simulink model "PID_quad_x_model"  (R2014b)
settings: Solver=ode45  StartTime=0.0  StopTime=30.0  RelTol=1e-3
libraries: simulink x5
settings Model: Creator=ghost  LastModifiedBy=ghost

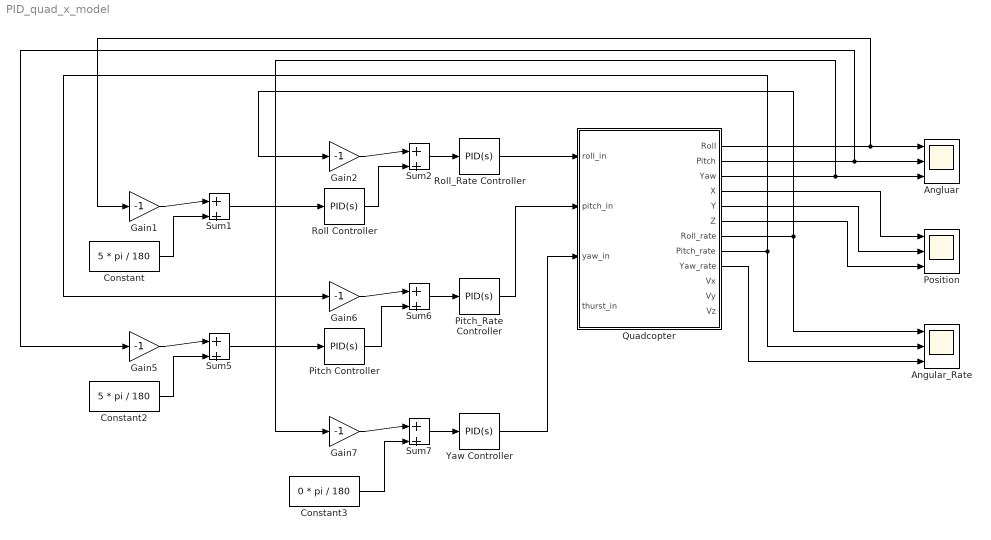
== system PID_quad_x_model ==
  Angluar : Scope  NumInputPorts=3
      settings: YMin=-5~-5~-5  YMax=5~5~5  SaveName=ScopeData2
  Angular_Rate : Scope  NumInputPorts=3
      settings: YMin=-5~-5~-5  YMax=5~5~5  SaveName=ScopeData3
  Constant : Constant  Value=5 * pi / 180
  Constant2 : Constant  Value=5 * pi / 180
  Constant3 : Constant  Value=0 * pi / 180
  Gain{1..2,5..7} (5 alike) : Gain  Gain=-1
  Pitch Controller : simulink/Continuous/PID Controller  Controller=PID  TimeDomain=Continuous-time  SampleTime=-1  IntegratorMethod=Forward Euler  FilterMethod=Forward Euler  Form=Parallel  P=10  I=0.05  D=0  N=100  InitialConditionSource=internal  InitialConditionForIntegrator=0  InitialConditionForFilter=0  ExternalReset=none  LimitOutput=off  UpperSaturationLimit=inf  LowerSaturationLimit=-inf  LinearizeAsGain=on  AntiWindupMode=none  Kb=1  TrackingMode=off  Kt=1  PParamMin=[]  PParamMax=[]  IParamMin=[]  IParamMax=[]  DParamMin=[]  DParamMax=[]  NParamMin=[]  NParamMax=[]  KbParamMin=[]  KbParamMax=[]  KtParamMin=[]  KtParamMax=[]  POutMin=[]  POutMax=[]  IOutMin=[]  IOutMax=[]  DOutMin=[]  DOutMax=[]  NOutMin=[]  NOutMax=[]  KbOutMin=[]  KbOutMax=[]  KtOutMin=[]  KtOutMax=[]  IntegratorOutMin=[]  IntegratorOutMax=[]  FilterOutMin=[]  FilterOutMax=[]  SumOutMin=[]  SumOutMax=[]  SumI1OutMin=[]  SumI1OutMax=[]  SumI2OutMin=[]  SumI2OutMax=[]  SumI3OutMin=[]  SumI3OutMax=[]  SumDOutMin=[]  SumDOutMax=[]  SaturationOutMin=[]  SaturationOutMax=[]  IntegratorContinuousStateAttributes=''  IntegratorStateMustResolveToSignalObject=off  IntegratorRTWStateStorageClass=Auto  FilterContinuousStateAttributes=''  FilterStateMustResolveToSignalObject=off  FilterRTWStateStorageClass=Auto  DifferentiatorICPrevScaledInput=0  DifferentiatorOutMin=[]  DifferentiatorOutMax=[]  UseFilter=on
  Pitch_Rate Controller : simulink/Continuous/PID Controller  Controller=PID  TimeDomain=Continuous-time  SampleTime=-1  IntegratorMethod=Forward Euler  FilterMethod=Forward Euler  Form=Parallel  P=1  I=0  D=0.1  N=100  InitialConditionSource=internal  InitialConditionForIntegrator=0  InitialConditionForFilter=0  ExternalReset=none  LimitOutput=off  UpperSaturationLimit=inf  LowerSaturationLimit=-inf  LinearizeAsGain=on  AntiWindupMode=none  Kb=1  TrackingMode=off  Kt=1  PParamMin=[]  PParamMax=[]  IParamMin=[]  IParamMax=[]  DParamMin=[]  DParamMax=[]  NParamMin=[]  NParamMax=[]  KbParamMin=[]  KbParamMax=[]  KtParamMin=[]  KtParamMax=[]  POutMin=[]  POutMax=[]  IOutMin=[]  IOutMax=[]  DOutMin=[]  DOutMax=[]  NOutMin=[]  NOutMax=[]  KbOutMin=[]  KbOutMax=[]  KtOutMin=[]  KtOutMax=[]  IntegratorOutMin=[]  IntegratorOutMax=[]  FilterOutMin=[]  FilterOutMax=[]  SumOutMin=[]  SumOutMax=[]  SumI1OutMin=[]  SumI1OutMax=[]  SumI2OutMin=[]  SumI2OutMax=[]  SumI3OutMin=[]  SumI3OutMax=[]  SumDOutMin=[]  SumDOutMax=[]  SaturationOutMin=[]  SaturationOutMax=[]  IntegratorContinuousStateAttributes=''  IntegratorStateMustResolveToSignalObject=off  IntegratorRTWStateStorageClass=Auto  FilterContinuousStateAttributes=''  FilterStateMustResolveToSignalObject=off  FilterRTWStateStorageClass=Auto  DifferentiatorICPrevScaledInput=0  DifferentiatorOutMin=[]  DifferentiatorOutMax=[]  UseFilter=on
  Position : Scope  NumInputPorts=3
      settings: YMin=-5~-5~-5  YMax=5~5~5  SaveName=ScopeData4
  Quadcopter : Subsystem
  Roll Controller : simulink/Continuous/PID Controller  Controller=PID  TimeDomain=Continuous-time  SampleTime=-1  IntegratorMethod=Forward Euler  FilterMethod=Forward Euler  Form=Parallel  P=10  I=0.05  D=0  N=100  InitialConditionSource=internal  InitialConditionForIntegrator=0  InitialConditionForFilter=0  ExternalReset=none  LimitOutput=off  UpperSaturationLimit=inf  LowerSaturationLimit=-inf  LinearizeAsGain=on  AntiWindupMode=none  Kb=1  TrackingMode=off  Kt=1  PParamMin=[]  PParamMax=[]  IParamMin=[]  IParamMax=[]  DParamMin=[]  DParamMax=[]  NParamMin=[]  NParamMax=[]  KbParamMin=[]  KbParamMax=[]  KtParamMin=[]  KtParamMax=[]  POutMin=[]  POutMax=[]  IOutMin=[]  IOutMax=[]  DOutMin=[]  DOutMax=[]  NOutMin=[]  NOutMax=[]  KbOutMin=[]  KbOutMax=[]  KtOutMin=[]  KtOutMax=[]  IntegratorOutMin=[]  IntegratorOutMax=[]  FilterOutMin=[]  FilterOutMax=[]  SumOutMin=[]  SumOutMax=[]  SumI1OutMin=[]  SumI1OutMax=[]  SumI2OutMin=[]  SumI2OutMax=[]  SumI3OutMin=[]  SumI3OutMax=[]  SumDOutMin=[]  SumDOutMax=[]  SaturationOutMin=[]  SaturationOutMax=[]  IntegratorContinuousStateAttributes=''  IntegratorStateMustResolveToSignalObject=off  IntegratorRTWStateStorageClass=Auto  FilterContinuousStateAttributes=''  FilterStateMustResolveToSignalObject=off  FilterRTWStateStorageClass=Auto  DifferentiatorICPrevScaledInput=0  DifferentiatorOutMin=[]  DifferentiatorOutMax=[]  UseFilter=on
  Roll_Rate Controller : simulink/Continuous/PID Controller  Controller=PID  TimeDomain=Continuous-time  SampleTime=-1  IntegratorMethod=Forward Euler  FilterMethod=Forward Euler  Form=Parallel  P=1  I=0  D=0.1  N=100  InitialConditionSource=internal  InitialConditionForIntegrator=0  InitialConditionForFilter=0  ExternalReset=none  LimitOutput=off  UpperSaturationLimit=inf  LowerSaturationLimit=-inf  LinearizeAsGain=on  AntiWindupMode=none  Kb=1  TrackingMode=off  Kt=1  PParamMin=[]  PParamMax=[]  IParamMin=[]  IParamMax=[]  DParamMin=[]  DParamMax=[]  NParamMin=[]  NParamMax=[]  KbParamMin=[]  KbParamMax=[]  KtParamMin=[]  KtParamMax=[]  POutMin=[]  POutMax=[]  IOutMin=[]  IOutMax=[]  DOutMin=[]  DOutMax=[]  NOutMin=[]  NOutMax=[]  KbOutMin=[]  KbOutMax=[]  KtOutMin=[]  KtOutMax=[]  IntegratorOutMin=[]  IntegratorOutMax=[]  FilterOutMin=[]  FilterOutMax=[]  SumOutMin=[]  SumOutMax=[]  SumI1OutMin=[]  SumI1OutMax=[]  SumI2OutMin=[]  SumI2OutMax=[]  SumI3OutMin=[]  SumI3OutMax=[]  SumDOutMin=[]  SumDOutMax=[]  SaturationOutMin=[]  SaturationOutMax=[]  IntegratorContinuousStateAttributes=''  IntegratorStateMustResolveToSignalObject=off  IntegratorRTWStateStorageClass=Auto  FilterContinuousStateAttributes=''  FilterStateMustResolveToSignalObject=off  FilterRTWStateStorageClass=Auto  DifferentiatorICPrevScaledInput=0  DifferentiatorOutMin=[]  DifferentiatorOutMax=[]  UseFilter=on
  Sum{1..2,5..7} (5 alike) : Sum  Inputs=|++
  Yaw Controller : simulink/Continuous/PID Controller  Controller=PID  TimeDomain=Continuous-time  SampleTime=-1  IntegratorMethod=Forward Euler  FilterMethod=Forward Euler  Form=Parallel  P=1  I=0  D=1.25  N=100  InitialConditionSource=internal  InitialConditionForIntegrator=0  InitialConditionForFilter=0  ExternalReset=none  LimitOutput=off  UpperSaturationLimit=inf  LowerSaturationLimit=-inf  LinearizeAsGain=on  AntiWindupMode=none  Kb=1  TrackingMode=off  Kt=1  PParamMin=[]  PParamMax=[]  IParamMin=[]  IParamMax=[]  DParamMin=[]  DParamMax=[]  NParamMin=[]  NParamMax=[]  KbParamMin=[]  KbParamMax=[]  KtParamMin=[]  KtParamMax=[]  POutMin=[]  POutMax=[]  IOutMin=[]  IOutMax=[]  DOutMin=[]  DOutMax=[]  NOutMin=[]  NOutMax=[]  KbOutMin=[]  KbOutMax=[]  KtOutMin=[]  KtOutMax=[]  IntegratorOutMin=[]  IntegratorOutMax=[]  FilterOutMin=[]  FilterOutMax=[]  SumOutMin=[]  SumOutMax=[]  SumI1OutMin=[]  SumI1OutMax=[]  SumI2OutMin=[]  SumI2OutMax=[]  SumI3OutMin=[]  SumI3OutMax=[]  SumDOutMin=[]  SumDOutMax=[]  SaturationOutMin=[]  SaturationOutMax=[]  IntegratorContinuousStateAttributes=''  IntegratorStateMustResolveToSignalObject=off  IntegratorRTWStateStorageClass=Auto  FilterContinuousStateAttributes=''  FilterStateMustResolveToSignalObject=off  FilterRTWStateStorageClass=Auto  DifferentiatorICPrevScaledInput=0  DifferentiatorOutMin=[]  DifferentiatorOutMax=[]  UseFilter=on
  wires:
  Sum1/1 -> Roll Controller/1
  Gain1/1 -> Sum1/1
  Constant/1 -> Sum1/2
  Roll_Rate Controller/1 -> Quadcopter/1(roll_in)
  Sum2/1 -> Roll_Rate Controller/1
  Gain2/1 -> Sum2/1
  Roll Controller/1 -> Sum2/2
  Quadcopter/7(Roll_rate) -> Angular_Rate/1, Gain2/1
  Quadcopter/1(Roll) -> Angluar/1, Gain1/1
  Quadcopter/2(Pitch) -> Angluar/2, Gain5/1
  Quadcopter/3(Yaw) -> Angluar/3, Gain7/1
  Sum5/1 -> Pitch Controller/1
  Gain5/1 -> Sum5/1
  Constant2/1 -> Sum5/2
  Sum6/1 -> Pitch_Rate Controller/1
  Gain6/1 -> Sum6/1
  Pitch Controller/1 -> Sum6/2
  Quadcopter/8(Pitch_rate) -> Angular_Rate/2, Gain6/1
  Pitch_Rate Controller/1 -> Quadcopter/2(pitch_in)
  Yaw Controller/1 -> Quadcopter/3(yaw_in)
  Sum7/1 -> Yaw Controller/1
  Gain7/1 -> Sum7/1
  Constant3/1 -> Sum7/2
  Quadcopter/9(Yaw_rate) -> Angular_Rate/3
  Quadcopter/4(X) -> Position/1
  Quadcopter/5(Y) -> Position/2
  Quadcopter/6(Z) -> Position/3

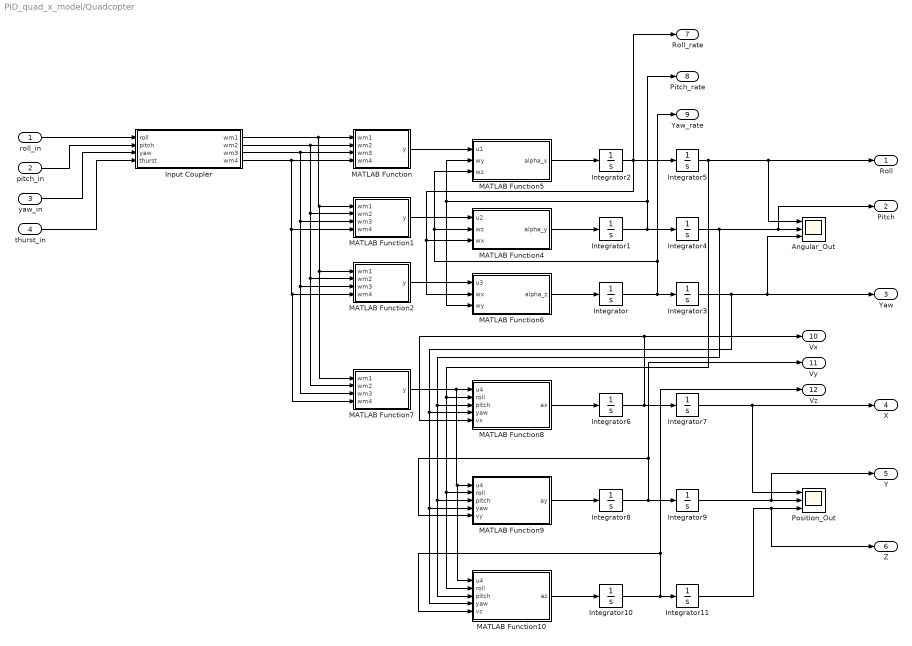
== system PID_quad_x_model/Quadcopter ==
  roll_in : Inport
  pitch_in : Inport  Port=2
  yaw_in : Inport  Port=3
  thurst_in : Inport  Port=4
  Angular_Out : Scope  NumInputPorts=3
      settings: YMin=-5~-5~-5  YMax=5~5~5
  Input Coupler : MATLAB Function  TreatAsAtomicUnit=on
  Integrator{,1..11} (12 alike) : Integrator
  MATLAB Function : MATLAB Function  TreatAsAtomicUnit=on
  MATLAB Function1 : MATLAB Function  TreatAsAtomicUnit=on
  MATLAB Function10 : MATLAB Function  TreatAsAtomicUnit=on
  MATLAB Function2 : MATLAB Function  TreatAsAtomicUnit=on
  MATLAB Function4 : MATLAB Function  TreatAsAtomicUnit=on
  MATLAB Function5 : MATLAB Function  TreatAsAtomicUnit=on
  MATLAB Function6 : MATLAB Function  TreatAsAtomicUnit=on
  MATLAB Function7 : MATLAB Function  TreatAsAtomicUnit=on
  MATLAB Function8 : MATLAB Function  TreatAsAtomicUnit=on
  MATLAB Function9 : MATLAB Function  TreatAsAtomicUnit=on
  "Position_Out " : Scope  NumInputPorts=3
      settings: YMin=-5~-5~-5  YMax=5~5~5
  Roll : Outport
  Pitch : Outport  Port=2
  Yaw : Outport  Port=3
  X : Outport  Port=4
  Y : Outport  Port=5
  Z : Outport  Port=6
  Roll_rate : Outport  Port=7
  Pitch_rate : Outport  Port=8
  Yaw_rate : Outport  Port=9
  Vx : Outport  Port=10
  Vy : Outport  Port=11
  Vz : Outport  Port=12
  wires:
  Input Coupler/1(wm1) -> MATLAB Function7/1(wm1), MATLAB Function2/1(wm1), MATLAB Function1/1(wm1), MATLAB Function/1(wm1)
  Input Coupler/2(wm2) -> MATLAB Function7/2(wm2), MATLAB Function2/2(wm2), MATLAB Function1/2(wm2), MATLAB Function/2(wm2)
  Input Coupler/3(wm3) -> MATLAB Function7/3(wm3), MATLAB Function2/3(wm3), MATLAB Function1/3(wm3), MATLAB Function/3(wm3)
  Input Coupler/4(wm4) -> MATLAB Function7/4(wm4), MATLAB Function2/4(wm4), MATLAB Function1/4(wm4), MATLAB Function/4(wm4)
  MATLAB Function1/1(y) -> MATLAB Function4/1(u2)
  MATLAB Function2/1(y) -> MATLAB Function6/1(u3)
  MATLAB Function6/1(alpha_z) -> Integrator/1
  Integrator/1 -> Integrator3/1, Yaw_rate/1, MATLAB Function5/3(wz), MATLAB Function4/2(wz)
  MATLAB Function5/1(alpha_x) -> Integrator2/1
  MATLAB Function4/1(alpha_y) -> Integrator1/1
  Integrator2/1 -> Integrator5/1, Roll_rate/1, MATLAB Function6/2(wx), MATLAB Function4/3(wx)
  Integrator3/1 -> MATLAB Function10/4(yaw), MATLAB Function9/4(yaw), MATLAB Function8/4(yaw), Yaw/1, Angular_Out/3
  Integrator4/1 -> Pitch/1, Angular_Out/2, MATLAB Function10/3(pitch), MATLAB Function9/3(pitch), MATLAB Function8/3(pitch)
  MATLAB Function/1(y) -> MATLAB Function5/1(u1)
  MATLAB Function8/1(ax) -> Integrator6/1
  Integrator6/1 -> Vx/1, MATLAB Function8/5(vx), Integrator7/1
  MATLAB Function7/1(y) -> MATLAB Function10/1(u4), MATLAB Function9/1(u4), MATLAB Function8/1(u4)
  MATLAB Function9/1(ay) -> Integrator8/1
  Integrator8/1 -> Vy/1, MATLAB Function9/5(vy), Integrator9/1
  MATLAB Function10/1(az) -> Integrator10/1
  Integrator5/1 -> MATLAB Function10/2(roll), MATLAB Function9/2(roll), MATLAB Function8/2(roll), Roll/1, Angular_Out/1
  Integrator7/1 -> X/1, "Position_Out "/1
  Integrator9/1 -> Y/1, "Position_Out "/2
  Integrator11/1 -> Z/1, "Position_Out "/3
  roll_in/1 -> Input Coupler/1(roll)
  pitch_in/1 -> Input Coupler/2(pitch)
  yaw_in/1 -> Input Coupler/3(yaw)
  thurst_in/1 -> Input Coupler/4(thurst)
  Integrator1/1 -> Pitch_rate/1, MATLAB Function5/2(wy), MATLAB Function6/3(wy), Integrator4/1
  Integrator10/1 -> Vz/1, MATLAB Function10/5(vz), Integrator11/1

== matlab function PID_quad_x_model/Quadcopter/MATLAB Function1 ==
  data: wm1 input; y output; wm2 input; wm3 input; wm4 input
function y = u2(wm1, wm2, wm3, wm4)
%#codegen

k1 = 3.1 * 10^-7;
y = k1 * (wm2^2 + wm4^2 - wm1^2 - wm3^2);
return;

== matlab function PID_quad_x_model/Quadcopter/MATLAB Function ==
  data: wm1 input; y output; wm2 input; wm3 input; wm4 input
function y = u1(wm1, wm2, wm3, wm4)
%#codegen

k1 = 3.1 * 10^-7;
y = k1 * (wm2^2 + wm3^2 - wm1^2 - wm4^2);
return;

== matlab function PID_quad_x_model/Quadcopter/MATLAB Function2 ==
  data: wm1 input; y output; wm2 input; wm3 input; wm4 input
function y = u3(wm1, wm2, wm3, wm4)
%#codegen

k2 = 3.1 * 10^-7;
y = k2 * (wm1^2 + wm2^2 - wm3^2 - wm4^2);
return;

== matlab function PID_quad_x_model/Quadcopter/Input Coupler ==
  data: roll input; wm1 output; pitch input; yaw input; thurst input; wm2 output; wm3 output; wm4 output
function [wm1, wm2, wm3, wm4] = input_coupler(roll, pitch, yaw, thurst)
%#codegen

% 控制耦合
% 输入是归一化的，-1~1

% 基础输入 1000
thurst_bias = 1407;

% 去归一化
roll  = roll  * 500;
pitch = pitch * 500;
yaw   = yaw   * 500;
thurst = thurst * 1000;

wm1 = thurst + thurst_bias - roll - pitch + yaw;
wm2 = thurst + thurst_bias + roll + pitch + yaw;
wm3 = thurst + thurst_bias + roll - pitch - yaw;
wm4 = thurst + thurst_bias - roll + pitch - yaw;


return;

== matlab function PID_quad_x_model/Quadcopter/MATLAB Function4 ==
  data: u2 input; wz input; alpha_y output; wx input
function alpha_y = calc_pitch_a(u2, wz, wx)
%#codegen

l = 0.25;
Jx = 0.033;
Jy = 0.033;
Jz = 0.061;

alpha_y = u2 * (sqrt(2) / 2) * l + (Jz - Jx) * wz * wx;
alpha_y = alpha_y / Jy;


return;

== matlab function PID_quad_x_model/Quadcopter/MATLAB Function5 ==
  data: u1 input; wy input; wz input; alpha_x output
function alpha_x = calc_roll_a(u1, wy, wz)
%#codegen

l = 0.25;
Jx = 0.033;
Jy = 0.033;
Jz = 0.061;

alpha_x = u1 * (sqrt(2) / 2) * l + (Jy - Jz) * wy * wz;
alpha_x = alpha_x / Jx;


return;

== matlab function PID_quad_x_model/Quadcopter/MATLAB Function6 ==
  data: u3 input; wx input; alpha_z output; wy input
function alpha_z = calc_yaw_a(u3, wx, wy)
%#codegen

l = 0.25;
Jx = 0.033;
Jy = 0.033;
Jz = 0.061;

alpha_z = u3 * l + (Jx - Jy) * wx * wy;
alpha_z = alpha_z / Jz;


return;

== matlab function PID_quad_x_model/Quadcopter/MATLAB Function7 ==
  data: wm1 input; y output; wm2 input; wm3 input; wm4 input
function y = u4(wm1, wm2, wm3, wm4)
%#codegen

k1 = 3.1 * 10^-7;
y = k1 * (wm1^2 + wm2^2 + wm3^2 + wm4^2);
return;

== matlab function PID_quad_x_model/Quadcopter/MATLAB Function8 ==
  data: u4 input; roll input; pitch input; ax output; yaw input; vx input
function ax = calc_ax(u4, roll, pitch, yaw, vx)
%#codegen
% roll  -> alpha
% pitch -> beta
% yaw   -> gamma

m  = 0.25;
g  = 9.81;
kf = 0;

ax = u4 * (sin(roll) * sin(yaw) + cos(roll) * sin(pitch) * cos(yaw));
ax = ax - kf * vx;
ax = ax / m;

return;

== matlab function PID_quad_x_model/Quadcopter/MATLAB Function9 ==
  data: u4 input; roll input; pitch input; ay output; yaw input; vy input
function ay = calc_ay(u4, roll, pitch, yaw, vy)
%#codegen
% roll  -> alpha
% pitch -> beta
% yaw   -> gamma

m  = 0.25;
g  = 9.81;
kf = 0;

ay = u4 * (-sin(roll) * cos(yaw) + cos(roll) * sin(pitch) * sin(yaw));
ay = ay - kf * vy;
ay = ay / m;

return;

== matlab function PID_quad_x_model/Quadcopter/MATLAB Function10 ==
  data: u4 input; roll input; pitch input; az output; yaw input; vz input
function az = calc_az(u4, roll, pitch, yaw, vz)
%#codegen
% roll  -> alpha
% pitch -> beta
% yaw   -> gamma

m  = 0.25;
g  = 9.81;
kf = 0;

az = u4 * (cos(roll) * cos(pitch));
az = az / m - g;

return;
